simulink library "PWM_ADCLib_For_MIL"  (R2025b)
settings: Solver=VariableStepAuto  StartTime=0.0  StopTime=10.0  RelTol=1e-3
libraries: simulink x1, eeGeneralControl x1
settings Model: Creator=ykamatan  LastModifiedBy=ykamatan

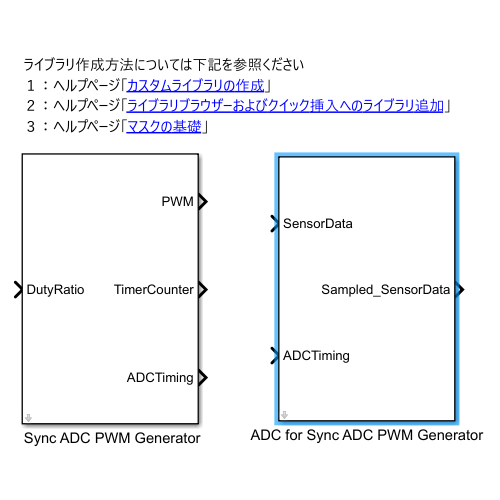
[thumbnail: Simulink's stored preview of the top-level diagram]
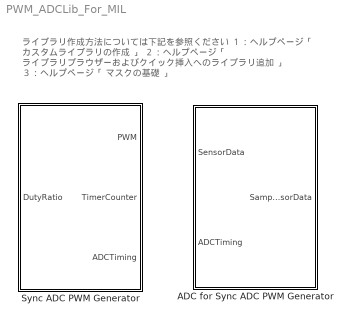
== system PWM_ADCLib_For_MIL ==
  note: ライブラリ作成方法については下記を参照ください
      | １：ヘルプページ「 カスタムライブラリの作成 」
      | ２：ヘルプページ「 ライブラリブラウザーおよびクイック挿入へのライブラリ追加 」
      | ３：ヘルプページ「 マスクの基礎 」
  " Sync ADC PWM Generator" : Subsystem  mask(Sync ADC PWM Generator){fsw=100000, PWM_Resolution=0.001, TimerCountMax=1000, DeadTimeRange=1, DeadTime=1e-08, MaxDuty=0.95, MinDuty=0.01, OutputVoltage=[]}
      mask prompts: fsw "スイッチング周波数 [Hz]"; PWM_Resolution "PWM解像度"; TimerCountMax "タイマカウント最大値"; DeadTimeRange "DeadTimeは最小ON時間の何倍に指定しますか:"; DeadTime "設定されたDeadTime[sec]"; MaxDuty "MaxDutyRatio"; MinDuty "MinDutyRatio"; OutputVoltage "PWM最大電圧"
      mask help:
      | 本サンプルライブラリはあくまでライブラリ化を実施した結果を示すもので、製品相当のライブラリと同等の品質検証を行ったものではありません。
      | あくまで参考までにご利用ください。
      | PWMキャリアと同期したADCを行うために作成されたPWMモジュールライブラリです。
      mask Help:
      | ■使いかた
      | 1．スイッチング周波数の指定
      | 2．PWM解像度の指定
      | 3．デットタイム幅の指定
      | 4．最大最小Dutyの指定
      | 5．出力されるPWM信号の最大値の指定
      | を行うことでPWMパルス生成が可能になります。
      | 
      | ■端子の解説
      | In:DutyRatio
      | Duty比を入力します。0～1の値を入力ください。
      | 
      | Out1:PWM
      | PWM波形信号が出力されます。
      | Simulink信号として出力されるため、Simscapeライブラリと接続する場合はSimulink-PS Converterライブラリを使用してSimscape信号に変換してください。
      | 
      | Out2:TimerCounter
      | ライブラリ内部でキャリア波形として利用しているタイマカウント値を出力します。
      | 
      | Out3:ADCTiming
      | キャリア波形の山の地点でADCがサンプリングするためのトリガ信号を出力します。
      | 本サンプルはキャリア波形形状の変更、谷でのサンプリング等タイミング変更に対応していません。
      | モデルの隠蔽化を行っていないので、内部モデルを編集することでそれらの変更に対応することは技術的に可能です。
      | 
      | ADC for Sync ADC PWM GeneratorのADCTiming端子に接続することでキャリアと動悸したサンプリングが可能です。
      mask DialogControl DescGroupVar Prompt: PWM Generatorパラメータ
      mask DialogControl Control2 Prompt: 1.スイッチング周波数を整数で入力ください。
      mask DialogControl fsw Tooltip: スイッチング周波数を指定ください。
      mask DialogControl Control3 Prompt: 2．シミュレーションで表現するPWM分解能を入力ください。例えばPWMのON/OFFの切り替え点をスイッチング周期あたり1000段階で表現したい場合はその逆数である0.001を入力します。
      mask DialogControl PWM_Resolution Tooltip: シミュレーションで表現するPWM分解能を入力ください。例えばPWMのON/OFFの切り替え点をスイッチング周期あたり1000段階で表現したい場合はその逆数である0.001を入力します。
      mask DialogControl Control7 Prompt: PWM解像度が指定されることでPWMキャリア波形を作成するタイマカウントの最大値が決定されます。なお、このサンプルはキャリア波形は三角波で固定となります。
      mask DialogControl Control5 Prompt: 3.デットタイムを指定します。シミュレーションではPWM解像度によって表現可能なパルス幅の最小単位が決定されます。最小Duty時間はToff=1/fsw*PWM_Resolution[sec]となり、この時間の倍数しかDeatTimeを指定できません。このダイアログでは最小OFF時間の何倍をデットタイムとして指定するか設定します。
      mask DialogControl Control4 Prompt: 4.最大最小のDuty時間を設定します
      mask DialogControl Control6 Prompt: このブロックのPWM端子から出力されるPWMパルス信号の最大電圧を指定します。仮に15を指定するとPWM端子から出力されるパルス信号はOFF時は０、ON時は15を出力します。
      mask DialogControl Instruction Prompt: 本サンプルライブラリについて
      mask DialogControl Control8 Prompt: 本サンプルライブラリはあくまでライブラリ化を実施した結果を示すもので、製品相当のライブラリと同等の品質検証を行ったものではありません。あくまで参考までにご利用ください。
  ADC for Sync ADC PWM Generator : Subsystem  mask(ADC for Sync ADC PWM Generator){ADC_QuantBit=12, QuantResolution=0.00024414, MaxRange=50, MinRange=-50, QuantUnit=0.024414}
      mask prompts: ADC_QuantBit "ADC量子化ビット数"; QuantResolution "量子解像度"; MaxRange "最大レンジ"; MinRange "最小レンジ"; QuantUnit "サンプル可能な最小刻み幅"
      mask help:
      | 本サンプルライブラリはあくまでライブラリ化を実施した結果を示すもので、製品相当のライブラリと同等の品質検証を行ったものではありません。
      | あくまで参考までにご利用ください。
      | PWMキャリアと同期したADCを行うために作成されたADCモジュールライブラリです。
      |
      | シンプルなADCの挙動をMILシミュレーションで表現します。
      mask Help:
      | ■使いかた
      | 1．ADC量子化ビット数
      | 2．サンプリングする値の最大・最小値
      | を行うことでPWMパルス生成が可能になります。
      | 
      | ■端子の解説
      | In1:SensorData
      | ADCでサンプリングしたいセンサデータを入力します。
      | 
      | In2:ADCTiming
      |  Sync ADC PWM GeneratorのADCTiming端子をこちらの端子に接続することで、
      | タイマカウントの山のタイミングでサンプリング可能になります。
      | 
      | Out:Sampled_SensorData
      | ADCによってサンプリングされた値が出力されます。
      mask DialogControl DescGroupVar Prompt: パラメータの設定
      mask DialogControl DescTextVar Prompt: 1．ADC量子化ビット指定
      mask DialogControl Control2 Prompt: 2．サンプル値最大最小値指定

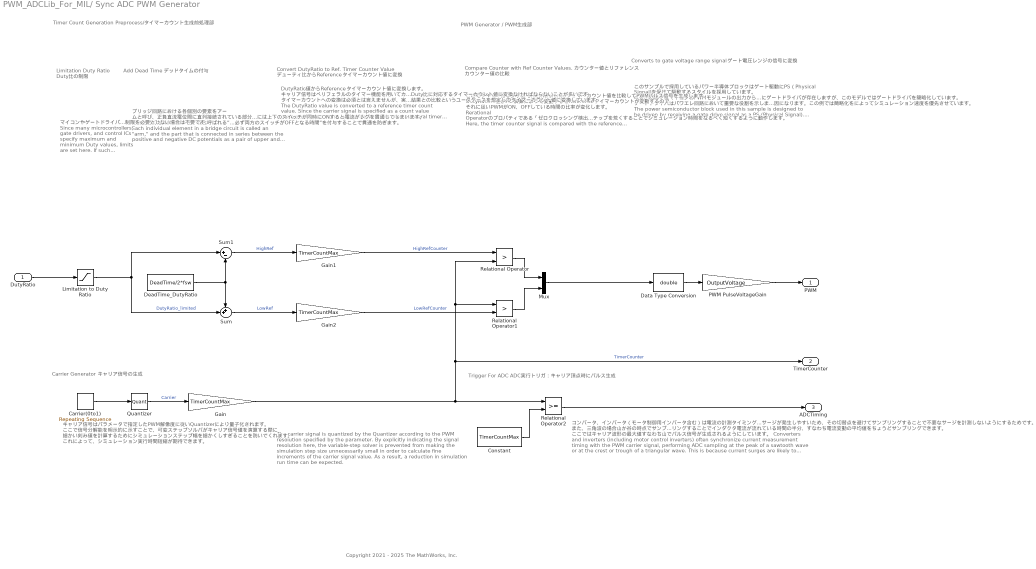
== system PWM_ADCLib_For_MIL/ Sync ADC PWM Generator ==
  note: The carrier signal is quantized by the Quantizer according to the PWM resolution specified by the parameter.
      | By explicitly indicating the signal resolution here, the variable-step solver is prevented from making the simulation step size unnecessarily small in order to calculate fine increments of the carrier signal value.
      | As a result, a reduction in simulation run time can be expected.
  note: Compare Counter with Ref Counter Values.
      | カウンター値とリファレンス カウンター値の比較
  note: Converts to gate voltage range signal
      | ゲート電圧レンジの信号に変換
  note: Carrier Generator
      | キャリア信号の生成
  note: PWM Generator / PWM生成部
  note: Timer Count Generation Preprocess/タイマーカウント生成前処理部
  note: Limitation
      | Duty Ratio
      |
      | Duty比の制限
  note: キャリア信号はパラメータで指定したPWM解像度に従いQuantizerにより量子化されます。
      | ここで信号分解能を明示的に示すことで、可変ステップソルバがキャリア信号値を演算する際に
      | 細かい刻み値を計算するためにシミュレーションステップ幅を細かくしすぎることを防いでくれます。
      | これによって、シミュレーション実行時間短縮が期待できます。
  note: Trigger For ADC
      | ADC実行トリガ：キャリア頂点時にパルス生成
  note: Convert DutyRatio to　Ref. Timer Counter Value
      | デューティ比からReferenceタイマーカウント値に変換
  note: Copyright 2021 - 2025 The MathWorks, Inc.
  note: このサンプルで採用しているパワー半導体ブロックはゲート駆動にPS（Physical Signal)を受けて駆動するスタイルを採用しています。
      |
      | 本来の回路ではマイコンのPWMモジュールの出力からパワー半導体デバイスの間にゲートドライバが存在しますが、このモデルではゲートドライバを簡略化しています。
      |
      | ゲートドライバはパワエレ回路において重要な役割を示しますが、正確な挙動表現には細かいモデリングが必要になり、結果としてシミュレーション速度が低下する原因になります。この例では簡略化をによってシミュレーション速度を優先させています。
      |
      | The power semiconductor block used in this sample is designed to be driven by receiving a gate drive signal as a PS (Physical Signal).
      |
      | In an actual circuit, a gate driver exists between the microcontroller's PWM module output and the power semiconductor device, but in this model, the gate driver is simplified.
      |
      | Gate drivers play an important role in power electronics circuits, but accurately representing their behavior requires detailed modeling, which can lead to slower simulation speeds. In this example, the gate driver is simplified to prioritize simulation speed.
  note: Add Dead Time
      | デッドタイムの付与
  note: ここでタイマーカウンタ信号とReferenceタイマーカウント値を比較してPWMパルス信号を生成します。
      |
      | DutyRatio値がPID演算によって変動するとReferenceタイマーカウントが変動するので、
      | それに従いPWMがON、OFFしている時間の比率が変化します。
      | Rerational Operatorのプロパティである「ゼロクロッシング検出を有効にする」を有効にすることで、可変ステップソルバは比較によって値が変動するタイミングで細かくステップを刻み、そうでない箇所ではタイムステップを荒くすることでシミュレーション時間をなるべく短くするように動作します。
      |
      | Here, the timer counter signal is compared with the reference timer count value to generate the PWM pulse signal.
      |
      | When the DutyRatio value fluctuates due to PID calculation, the reference timer count also changes,
      | which in turn changes the ratio of the ON and OFF times of the PWM signal accordingly.
      | By enabling the "Enable zero-crossing detection" property of the Relational Operator, the variable-step solver will take finer steps at the timing when the comparison causes the value to change, and use coarser time steps elsewhere. This helps to minimize the simulation time as much as possible.
  note: DutyRatio値からReferenceタイマーカウント値に変換します。
      |
      | キャリア信号はペリフェラルのタイマー機能を用いてカウントアップ・カウントダウンによって生成されるカウント値として指定されるので、Duty値もまた、Duty比に対応するタイマーカウント値に変換なければならないことが多いです。
      | タイマーカウントへの変換は必須とは言えませんが、実機実験でのデバック結果との比較というユースケースを想定してタイマーカウント値に変換しています。
      |
      | The DutyRatio value is converted to a reference timer count value.
      |
      | Since the carrier signal is specified as a count value generated by counting up and down using the peripheral timer function,
      | the Duty value also often needs to be converted to a timer count value corresponding to the duty ratio.
      | Although conversion to a timer count is not strictly required, in this case, the DutyRatio is converted to a timer count value, assuming use cases such as comparison with debug results from actual hardware experiments.
  note: コンバータ、インバータ（モータ制御用インバータ含む）は電流の計測タイミングをPWMキャリア信号と同期させることが多く、ノコギリ波の頂点、もしくは三角波の山か谷のタイミングでADCのサンプリングを行います。これはPWMパルス電圧が切り替わる瞬間は電流サージが発生しやすいため、その切替点を避けてサンプリングすることで不要なサージを計測しないようにするためです。
      | また、三角波の場合山か谷の時点でサンプリングすることでインダクタ電流が流れている時間の半分、すなわち電流変動の平均値をちょうどサンプリングできます。
      | ここではキャリア波形の最大値すなわち山でパルス信号が生成されるようにしています。
      |
      | Converters and inverters (including motor control inverters) often synchronize current measurement timing with the PWM carrier signal, performing ADC sampling at the peak of a sawtooth wave or at the crest or trough of a triangular wave.
      | This is because current surges are likely to occur at the instant when the PWM pulse voltage switches, so sampling is performed away from these switching points to avoid measuring unnecessary surges.
      | Additionally, in the case of a triangular wave, sampling at the crest or trough allows you to sample exactly at the midpoint of the inductor current flow, that is, at the average value of the current fluctuation.
      |
      | In this example, the pulse signal is generated at the maximum value (the crest) of the carrier waveform.
  note: ブリッジ回路における各個別の要素をアー ムと呼び、正負直流電位間に直列接続されている部分を上下一組でレグと呼びます。今回回路に用いているハーフブリッジ回路は単一のレグに相当します。レグを駆動する際には上下のスイッチが同時にONすると電流がレグを貫通してしまいます。
      | それを防ぐためにデットタイムと呼ばれる”必ず両方のスイッチがOFFとなる時間”を付与することで貫通を防ぎます。
      |
      | Each individual element in a bridge circuit is called an "arm," and the part that is connected in series between the positive and negative DC potentials as a pair of upper and lower arms is called a "leg."
      | The half-bridge circuit used in this example corresponds to a single leg.
      | When driving a leg, if the upper and lower switches are turned ON at the same time, current will flow directly through the leg.
      | To prevent this, a period called "dead time"—during which both switches are definitely OFF—is added to avoid such direct current flow.
  note: マイコンやゲートドライバ、制御ICにはDutyの最大値、最小値が指定されているものも多いためここで制限を設けています。制限を必要としない場合は不要です。
      |
      | Since many microcontrollers, gate drivers, and control ICs specify maximum and minimum Duty values, limits are set here.
      | If such restrictions are not necessary, this limitation can be omitted.
  DutyRatio : Inport
  Carrier(0to1) : simulink/Sources/Repeating Sequence  rep_seq_t=[0 1/fsw/2 1/fsw]  rep_seq_y=[1 0 1]
  Constant : Constant  Value=TimerCountMax  OutDataTypeStr=uint16
  Data Type Conversion : DataTypeConversion  OutDataTypeStr=double  SaturateOnIntegerOverflow=off  RndMeth=Floor
  DeadTime_DutyRatio : Constant  Value=DeadTime/2*fsw  OutDataTypeStr=double
  Gain : Gain  Gain=TimerCountMax  OutDataTypeStr=double
  Gain1 : Gain  Gain=TimerCountMax
  Gain2 : Gain  Gain=TimerCountMax  OutDataTypeStr=double
  Limitation to Duty Ratio : Saturate  UpperLimit=MaxDuty  LowerLimit=MinDuty
  Mux : Mux  Inputs=2
  PWM PulseVoltageGain : Gain  Gain=OutputVoltage
  Quantizer : Quantizer  QuantizationInterval=PWM_Resolution
  Relational Operator : RelationalOperator  Operator=>  OutDataTypeStr=boolean  RndMeth=Simplest
  Relational Operator1 : RelationalOperator  Operator=>  OutDataTypeStr=boolean  RndMeth=Simplest
  Relational Operator2 : RelationalOperator  OutDataTypeStr=boolean  RndMeth=Simplest  InputSameDT=off
  Sum : Sum  Inputs=++|
  Sum1 : Sum  Inputs=|+-
  PWM : Outport
  TimerCounter : Outport  Port=2
  ADCTiming : Outport  Port=3
  wires:
  Gain1/1 -> Relational Operator/1  "HighRefCounter"
  DeadTime_DutyRatio/1 -> Sum1/2, Sum/1
  Gain2/1 -> Relational Operator1/2  "LowRefCounter"
  Sum1/1 -> Gain1/1  "HighRef"
  Limitation to Duty Ratio/1 -> Sum/2, Sum1/1  "DutyRatio_limited"
  Relational Operator1/1 -> Mux/2
  Gain/1 -> Relational Operator2/1, TimerCounter/1, Relational Operator1/1, Relational Operator/2  "TimerCounter"
  PWM PulseVoltageGain/1 -> PWM/1
  DutyRatio/1 -> Limitation to Duty Ratio/1
  Mux/1 -> Data Type Conversion/1
  Quantizer/1 -> Gain/1  "Carrier"
  Sum/1 -> Gain2/1  "LowRef"
  Constant/1 -> Relational Operator2/2
  Relational Operator2/1 -> ADCTiming/1
  Relational Operator/1 -> Mux/1
  Data Type Conversion/1 -> PWM PulseVoltageGain/1
  Carrier(0to1)/1 -> Quantizer/1

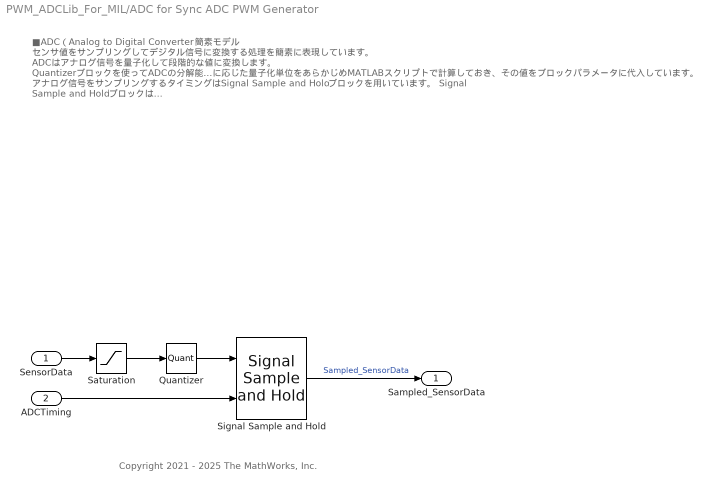
== system PWM_ADCLib_For_MIL/ADC for Sync ADC PWM Generator ==
  note: Copyright 2021 - 2025 The MathWorks, Inc.
  note: ■ADC（Analog to Digital Converter)簡素モデル
      | センサ値をサンプリングしてデジタル信号に変換する処理を簡素に表現しています。
      | ADCはアナログ信号を量子化して段階的な値に変換します。
      | Quantizerブロックを使ってADCの分解能に応じた量子化単位をあらかじめMATLABスクリプトで計算しておき、その値をブロックパラメータに代入しています。
      | アナログ信号をサンプリングするタイミングはSignal Sample and Holdブロックを用いています。
      | Signal Sample and Holdブロックは
      | Inにサンプリングしたい信号、Sにサンプリングタイミングを指定するパルス信号を入力することで、
      | そのタイミングでInの値をサンプリングし、それ以降次のパルスが入るまで値を保持します。
      |
      | ■Simplified ADC (Analog to Digital Converter) Model
      | This section provides a simplified representation of the process in which sensor values are sampled and converted into digital signals.
      | An ADC quantizes analog signals and converts them into discrete values.
      | The quantization unit corresponding to the ADC resolution is pre-calculated using a MATLAB script and entered as a block parameter in the Quantizer block.
      | The timing for sampling the analog signal is controlled using the Signal Sample and Hold block.
      | For the Signal Sample and Hold block, you input the signal you want to sample to the "u" port, and a pulse signal specifying the sampling timing to the "S" port.
      | At each pulse, the block samples the value of "u" and holds that value until the next pulse arrives.
  SensorData : Inport
  ADCTiming : Inport  Port=2
  Quantizer : Quantizer  QuantizationInterval=QuantUnit
  Saturation : Saturate  UpperLimit=MaxRange  LowerLimit=MinRange
  Signal Sample and Hold : eeGeneralControl/Signal Sample and Hold  LabelModeActiveChoice=Discrete  x0=0  Ts=-1
  Sampled_SensorData : Outport
  wires:
  Quantizer/1 -> Signal Sample and Hold/1
  Signal Sample and Hold/1 -> Sampled_SensorData/1  "Sampled_SensorData"
  ADCTiming/1 -> Signal Sample and Hold/2
  SensorData/1 -> Saturation/1
  Saturation/1 -> Quantizer/1
